simulink model "threelevel_12phase1"  (R2020b)
settings: Solver=FixedStepDiscrete  StartTime=0.0  StopTime=1  FixedStep=Ts_FEA  RelTol=1e-3
model workspace (MAT data in the model file):
  T_10kHz : Simulink.Parameter (value not decoded)
undefined symbols (not defined in the file): Cin, DiscIntNeverNeededParam, ESL, ESR, faif, Jm, kfeed_r, ki_n, kp_n, L, Ld, Line, Lq, ncmd_climb, ncmd_cruise, ncmd_run, ncmd_takeoff, p, Pcmd_climb, Pcmd_cruise, Pcmd_run, Pcmd_takeoff, Rs, Tcmd_run, Tcmd_start, Tcmd_time, time_climb, time_cruise, time_run, time_start, time_takeoff, Ts, Ts_Dead, Ts_FEA, Ts_speedloop, tswitch_climb, tswitch_takeoff, VDC, ws, zero_C1
libraries: powerlib x73, simulink x16, powerlib_meascontrol x16, slpidlib x13
(part 4 of 6)

== matlab function threelevel_12phase1/CurrentLoop/Subsystem/Subsystem/propose method1 ==
  data: PI input; r output; alpha input; beta input; phi input
function r = fcn(PI,alpha,beta,phi)

    M=sqrt(alpha^2+beta^2);
    alp_M  = alpha/M;
    beta_M = beta/M;

    M=1.1547*M;

    if(M<=1/sqrt(3)) 
        M3C= 0.1500*phi*phi*phi+0.0352*phi*phi+0.00783*phi+0.2609;
        M9C=-0.2472*phi*phi*phi-0.0606*phi*phi-0.01287*phi-0.3448;
        M3S= 0.3370*phi*phi+0.6254*phi;
        M9S=-0.0779*phi*phi-0.1659*phi;
    elseif(M<2/3)
        M3C=-3.6560+13.670*M-0.1007*phi-11.930*M*M+0.1374*M*phi+0.1620*phi*phi;
        M9C= 0.4058-3.4580*M+0.1805*phi+3.7340*M*M-0.2433*M*phi-0.2790*phi*phi;
        M3S= 0.7860-2.5180*M-0.6832*phi+2.0240*M*M+2.2250*M*phi+0.3401*phi*phi;
        M9S= 0.0754-0.2625*M+0.4331*phi+0.2243*M*M-1.0250*M*phi-0.0853*phi*phi;
    elseif(M<=0.84)
        M3C= 2.9760-6.4130*M-0.1877*phi+3.2850*M*M+0.2125*M*phi+0.2343*phi*phi;
        M9C=-0.4525-0.6800*M+0.3454*phi+1.4460*M*M-0.3967*M*phi-0.3939*phi*phi;
        M3S= 0.9292-2.4140*M-1.6830*phi+1.5730*M*M+3.5520*M*phi+0.5395*phi*phi;
        M9S=-0.2812+0.7235*M+0.7560*phi-0.4670*M*M-1.4380*M*phi-0.1593*phi*phi; 
    elseif(M<=1.16)
        M3C=-2.1320+5.5280*M-0.3833*phi-3.7000*M*M+0.4197*M*phi+0.2730*phi*phi;
        M9C= 1.0050-3.4350*M+0.5720*phi+2.6570*M*M-0.6220*M*phi-0.4592*phi*phi;
        M3S= 3.3150-7.2060*M-5.4830*phi+3.9060*M*M+8.0500*M*phi+0.4916*phi*phi;
        M9S=-0.9551+2.0770*M+1.5220*phi-1.1270*M*M-2.3370*M*phi-0.1548*phi*phi;
    else
        M3C = 0;
        M9C = 0;
        M3S = 0;
        M9S = 0;
    end

    cos_3 = -3*alp_M + 4*alp_M*alp_M*alp_M;
    cos_9 = -3*cos_3 + 4*cos_3*cos_3*cos_3;
    sin_3 =  3*beta_M - 4*beta_M*beta_M*beta_M;
    sin_9 =  3*sin_3  - 4*sin_3*sin_3*sin_3;
    
    r=M3C*cos_3+ M9C*cos_9+ M3S*sin_3+ M9S*sin_9+PI;
end

== matlab function threelevel_12phase1/CurrentLoop/NTSV_9_nearest ==
  data: Alpha input; Beta input; Ta1 output; Ta2 output; Tb1 output; Tb2 output; Tc1 output; Tc2 output; r input; VecSector1 output
function [Ta1,Ta2,Tb1,Tb2,Tc1,Tc2,VecSector1]  = fcn(Alpha,Beta,r)
temp1=Beta;
temp2=0.8660254*Alpha+Beta*0.5;
temp3=temp2-temp1;%0.8660254*Alpha-0.5beta
%temp1+temp2 0.8660254*Alpha+1.5beta
%temp3+temp2 2*0.8660254*Alpha
%temp1-temp3 -0.8660254*Alpha+1.5beta
VecSector1=3;
VecSector2=1;
VecSector3=0;
if temp2>0
    VecSector1=VecSector1-1;
end
if temp3>0
    VecSector1=VecSector1-1;
end
if temp1<0
    VecSector1=7-VecSector1;
end 
switch VecSector1
    case {1,4}  
       if(abs(temp2)>0.5)
           VecSector2=VecSector2+1;
           if(abs(temp3)<0.5)
               VecSector2=VecSector2+1;
               if(abs(temp1)>0.5)
                   VecSector2=VecSector2+1;
               end
           end
       end
       if(temp1<temp3)
           VecSector3=1;
       else
           VecSector3=2;
       end
    case {2,5}
       if(abs(temp1)>0.5)
           VecSector2=VecSector2+1;
           if(abs(temp2)<0.5)
               VecSector2=VecSector2+1;
               if(abs(temp3)>0.5)
                   VecSector2=VecSector2+1;
               end
           end
       end
       if(temp2+temp3>0)
          VecSector3=1;
       else
           VecSector3=2;
       end 
    case {3,6}
       if(abs(temp3)>0.5)
           VecSector2=VecSector2+1;
           if(abs(temp1)<0.5)
               VecSector2=VecSector2+1;
               if(abs(temp2)>0.5)
                   VecSector2=VecSector2+1;
               end
           end
       end
       if(temp1+temp2>0)
          VecSector3=1;
       else
           VecSector3=2;
       end 
    otherwise
        VecSector1=0;
        VecSector2=0;
end

switch VecSector1
    case 1
        Ta1=temp2;
        Ta2=1;
        Tc1=0;
        Tc2=1-temp2;
        switch VecSector2
            case 1
                Tb1=temp1;
                Tb2=1-temp3;
            case 2
                Tb1=0;
                Tb2=1+temp1-temp3;
            case 3
                Tb1=0.5-temp3;
                Tb2=0.5+temp1;
            case 4
                Tb1=temp1-temp3;
                Tb2=1;
            otherwise
                Tb1=0;
                Tb2=1;
        end
        if(VecSector3==1)
            Ta1=Ta1+Tc2*r;
            Tb2=Tb2+Tc2*r;
            Tc2=Tc2+Tc2*r;
        else
            Ta1=Ta1+Tc2*r;
            Tb1=Tb1+Tc2*r;
            Tc2=Tc2+Tc2*r;
        end
%--------------------------------------------------%
    case 2
        Tb1=temp1;
        Tb2=1;
        Tc1=0;
        Tc2=1-temp1;
        switch VecSector2
            case 1
                Ta1=temp2;
                Ta2=1+temp3;
            case 2
                Ta1=temp2+temp3;
                Ta2=1;
            case 3
                Ta1=0.5+temp3;
                Ta2=0.5+temp2;
            case 4
                Ta1=0;
                Ta2=1+temp2+temp3;
            otherwise
                Ta1=0;
                Ta2=1;
        end
        if(VecSector3==1)
            Ta1=Ta1+Tc2*r;
            Tb1=Tb1+Tc2*r;
            Tc2=Tc2+Tc2*r;
        else
            Ta2=Ta2+Tc2*r;
            Tb1=Tb1+Tc2*r;
            Tc2=Tc2+Tc2*r;
        end
%--------------------------------------------------%
    case 3
        Ta1=0;
        Ta2=1+temp3;
        Tb1=-temp3;
        Tb2=1;
        switch VecSector2
            case 1
                Tc1=-temp2;
                Tc2=1-temp1;
            case 2
                Tc1=0;
                Tc2=1-temp1-temp2;
            case 3
                Tc1=0.5-temp1;
                Tc2=0.5-temp2;
            case 4
                Tc1=-temp1-temp2;
                Tc2=1;
            otherwise
                Tc1=0;
                Tc2=1;
        end
        if(VecSector3==1)
            Tb1=Tb1+Ta2*r;
            Tc2=Tc2+Ta2*r;
            Ta2=Ta2+Ta2*r;
        else
            Tb1=Tb1+Ta2*r;
            Tc1=Tc1+Ta2*r;
            Ta2=Ta2+Ta2*r;
        end
%--------------------------------------------------%
    case 4
        Ta1=0;
        Ta2=1+temp2;
        Tc1=-temp2;
        Tc2=1;
        switch VecSector2
            case 1
                Tb1=-temp3;
                Tb2=1+temp1;
            case 2
                Tb1=temp1-temp3;
                Tb2=1;
            case 3
                Tb1=0.5+temp1;
                Tb2=0.5-temp3;
            case 4
                Tb1=0;
                Tb2=1+temp1-temp3;
            otherwise
                Tb1=0;
                Tb2=1;
        end
        if(VecSector3==1)
            Tb1=Tb1+Ta2*r;
            Tc1=Tc1+Ta2*r;
            Ta2=Ta2+Ta2*r;
        else
            Tb2=Tb2+Ta2*r;
            Tc1=Tc1+Ta2*r;
            Ta2=Ta2+Ta2*r;
        end
%--------------------------------------------------%
    case 5
        Tb1=0;
        Tb2=1+temp1;
        Tc1=-temp1;
        Tc2=1;
        switch VecSector2
            case 1
                Ta1=temp3;
                Ta2=1+temp2;
            case 2
                Ta1=0;
                Ta2=1+temp2+temp3;
            case 3
                Ta1=0.5+temp2;
                Ta2=0.5+temp3;
            case 4
                Ta1=temp2+temp3;
                Ta2=1;
            otherwise
                Ta1=0;
                Ta2=1;
        end
        if(VecSector3==1)
            Ta2=Ta2+Tb2*r;
            Tc1=Tc1+Tb2*r;
            Tb2=Tb2+Tb2*r;
        else
            Ta1=Ta1+Tb2*r;
            Tc1=Tc1+Tb2*r;
            Tb2=Tb2+Tb2*r;
        end
%--------------------------------------------------%
    case 6
        Ta1=temp3;
        Ta2=1;
        Tb1=0;
        Tb2=1-temp3;
        switch VecSector2
            case 1
                Tc1=-temp1;
                Tc2=1-temp2;
            case 2
                Tc1=-temp1-temp2;
                Tc2=1;
            case 3
                Tc1=0.5-temp2;
                Tc2=0.5-temp1;
            case 4
                Tc1=0;
                Tc2=1-temp1-temp2;
            otherwise
                Tc1=0;
                Tc2=1;
        end
        if(VecSector3==1)
            Ta1=Ta1+Tb2*r;
            Tc1=Tc1+Tb2*r;
            Tb2=Tb2+Tb2*r;
        else
            Ta1=Ta1+Tb2*r;
            Tc2=Tc2+Tb2*r;
            Tb2=Tb2+Tb2*r;
        end
%--------------------------------------------------%
    otherwise
        Ta1=0;
        Ta2=1;
        Tb1=0;
        Tb2=1;
        Tc1=0;
        Tc2=1;
end

== matlab function threelevel_12phase1/CurrentLoop/双载波SVPWM2 ==
  data: Alpha input; Beta input; Ta1 output; Ta2 output; Tb1 output; Tb2 output; Tc1 output; Tc2 output; r input; VecSector1 output
function [Ta1,Ta2,Tb1,Tb2,Tc1,Tc2,VecSector1]  = fcn(Alpha,Beta,r)
temp1=Beta;
temp2=0.8660254*Alpha+Beta*0.5;
temp3=temp2-temp1;%0.8660254*Alpha-0.5beta
%temp1+temp2 0.8660254*Alpha+1.5beta
%temp3+temp2 2*0.8660254*Alpha
%temp1-temp3 -0.8660254*Alpha+1.5beta
VecSector1=3;

x=sqrt(3)*Beta;
y=sqrt(3)*(sqrt(3)/2*Alpha+0.5*Beta);
z=sqrt(3)*(-sqrt(3)/2*Alpha+0.5*Beta);

if temp2>0
    VecSector1=VecSector1-1;
end
if temp3>0
    VecSector1=VecSector1-1;
end
if temp1<0
    VecSector1=7-VecSector1;
end 

switch VecSector1
    case 1
        TL=-z;
        TH=x;
        T07=1-TL-TH;
%--------------------------------------------------%
    case 2
        TL=z;
        TH=y;
        T07=1-TL-TH;
%--------------------------------------------------%
    case 3
        TL=x;
        TH=-y;
        T07=1-TL-TH;
%--------------------------------------------------%
    case 4
        TL=-x;
        TH=z;
        T07=1-TL-TH;
%--------------------------------------------------%
    case 5
        TL=-y;
        TH=-z;
        T07=1-TL-TH;
%--------------------------------------------------%
    case 6
        TL=y;
        TH=-x;
        T07=1-TL-TH;
%--------------------------------------------------%
    otherwise
        T07=0;
        TL=0;
        TH=0;
end

T7=T07*(1+r)/2;
Ta=0;
Tb=0;
Tc=0;

switch VecSector1
    case 1
    Ta=TH+TL+T7;
    Tb=TH+T7;
    Tc=T7;
    case  2
    Ta=TH+T7;
    Tb=TH+TL+T7;
    Tc=T7;
    case  3
    Ta=T7;
    Tb=TH+TL+T7;
    Tc=TH+T7;
    case  4
    Ta=T7;
    Tb=TH+T7;
    Tc=TH+TL+T7;
    case  5
    Ta=TH+T7;
    Tb=T7;
    Tc=TH+TL+T7;
    case  6
    Ta=TH+TL+T7;
    Tb=T7;
    Tc=TH+T7;     
end

Ta=Ta*2-1;
Tb=Tb*2-1;
Tc=Tc*2-1;

Ta1=Ta*(Ta>0);
Ta1=1-Ta1;
Ta2=Ta*(Ta<0);
Ta2=Ta2+1;
Ta2=1-Ta2;
Tb1=Tb*(Tb>0);
Tb1=1-Tb1;
Tb2=Tb*(Tb<0);
Tb2=Tb2+1;
Tb2=1-Tb2;
Tc1=Tc*(Tc>0);
Tc1=1-Tc1;
Tc2=Tc*(Tc<0);
Tc2=Tc2+1;
Tc2=1-Tc2;

== matlab function threelevel_12phase1/CurrentLoop/Subsystem2/Subsystem/propose method1 ==
  data: PI input; r output; alpha input; beta input; phi input
function r = fcn(PI,alpha,beta,phi)

    M=sqrt(alpha^2+beta^2);
    alp_M  = alpha/M;
    beta_M = beta/M;

    M=1.1547*M;

    if(M<=1/sqrt(3)) 
        M3C= 0.1500*phi*phi*phi+0.0352*phi*phi+0.00783*phi+0.2609;
        M9C=-0.2472*phi*phi*phi-0.0606*phi*phi-0.01287*phi-0.3448;
        M3S= 0.3370*phi*phi+0.6254*phi;
        M9S=-0.0779*phi*phi-0.1659*phi;
    elseif(M<2/3)
        M3C=-3.6560+13.670*M-0.1007*phi-11.930*M*M+0.1374*M*phi+0.1620*phi*phi;
        M9C= 0.4058-3.4580*M+0.1805*phi+3.7340*M*M-0.2433*M*phi-0.2790*phi*phi;
        M3S= 0.7860-2.5180*M-0.6832*phi+2.0240*M*M+2.2250*M*phi+0.3401*phi*phi;
        M9S= 0.0754-0.2625*M+0.4331*phi+0.2243*M*M-1.0250*M*phi-0.0853*phi*phi;
    elseif(M<=0.84)
        M3C= 2.9760-6.4130*M-0.1877*phi+3.2850*M*M+0.2125*M*phi+0.2343*phi*phi;
        M9C=-0.4525-0.6800*M+0.3454*phi+1.4460*M*M-0.3967*M*phi-0.3939*phi*phi;
        M3S= 0.9292-2.4140*M-1.6830*phi+1.5730*M*M+3.5520*M*phi+0.5395*phi*phi;
        M9S=-0.2812+0.7235*M+0.7560*phi-0.4670*M*M-1.4380*M*phi-0.1593*phi*phi; 
    elseif(M<=1.16)
        M3C=-2.1320+5.5280*M-0.3833*phi-3.7000*M*M+0.4197*M*phi+0.2730*phi*phi;
        M9C= 1.0050-3.4350*M+0.5720*phi+2.6570*M*M-0.6220*M*phi-0.4592*phi*phi;
        M3S= 3.3150-7.2060*M-5.4830*phi+3.9060*M*M+8.0500*M*phi+0.4916*phi*phi;
        M9S=-0.9551+2.0770*M+1.5220*phi-1.1270*M*M-2.3370*M*phi-0.1548*phi*phi;
    else
        M3C = 0;
        M9C = 0;
        M3S = 0;
        M9S = 0;
    end

    cos_3 = -3*alp_M + 4*alp_M*alp_M*alp_M;
    cos_9 = -3*cos_3 + 4*cos_3*cos_3*cos_3;
    sin_3 =  3*beta_M - 4*beta_M*beta_M*beta_M;
    sin_9 =  3*sin_3  - 4*sin_3*sin_3*sin_3;
    
    r=M3C*cos_3+ M9C*cos_9+ M3S*sin_3+ M9S*sin_9+PI;
end

== matlab function threelevel_12phase1/PMSM/MATLAB Function2 ==
  data: I input; Tem output; faif parameter; p parameter; fai_d1 output; fai_d2 output; fai_d3 output; fai_d4 output; fai_q1 output; fai_q2 output; fai_q3 output; fai_q4 output; Temp_L input
function [Tem,fai_d1,fai_d2,fai_d3,fai_d4,fai_q1,fai_q2,fai_q3,fai_q4] = Tem(I,faif,p,Temp_L)

% Temp_fai = Temp_L * I;
Temp_fai=Temp_L;
fai_d1=Temp_fai(1,1)+faif;
fai_d2=Temp_fai(3,1)+faif;
fai_d3=Temp_fai(5,1)+faif;
fai_d4=Temp_fai(7,1)+faif;
fai_q1=Temp_fai(2,1);
fai_q2=Temp_fai(4,1);
fai_q3=Temp_fai(6,1);
fai_q4=Temp_fai(8,1);
Tem1=3/2*p*(fai_d1*I(2,1)-fai_q1*I(1,1));
Tem2=3/2*p*(fai_d2*I(4,1)-fai_q2*I(3,1));
Tem3=3/2*p*(fai_d3*I(6,1)-fai_q3*I(5,1));
Tem4=3/2*p*(fai_d4*I(8,1)-fai_q4*I(7,1));
Tem=Tem1+Tem2+Tem3+Tem4;

== matlab function threelevel_12phase1/CurrentLoop/Subsystem3/NTSV_7_nearest ==
  data: Alpha input; Beta input; Ta1 output; Ta2 output; Tb1 output; Tb2 output; Tc1 output; Tc2 output; r input; r output
function [Ta1,Ta2,Tb1, Tb2,Tc1,Tc2,r]  = fcn(Alpha,Beta,r)
temp1=Beta;
temp2=0.8660254*Alpha+Beta*0.5;
temp3=temp2-temp1;%0.8660254*Alpha-0.5beta
VecSector1=3;
VecSector2=1;
VecSector3=0;
if temp2>0
    VecSector1=VecSector1-1;
end
if temp3>0
    VecSector1=VecSector1-1;
end
if temp1<0
    VecSector1=7-VecSector1;
end 
switch VecSector1
    case {1,4}  
       if(abs(temp2)>0.5)
           VecSector2=VecSector2+1;
           if(abs(temp3)<0.5)
               VecSector2=VecSector2+1;
               if(abs(temp1)>0.5)
                   VecSector2=VecSector2+1;
               end
           end
       end
       if(temp1<temp3)
           VecSector3=1;
       else
           VecSector3=2;
       end
    case {2,5}
       if(abs(temp1)>0.5)
           VecSector2=VecSector2+1;
           if(abs(temp2)<0.5)
               VecSector2=VecSector2+1;
               if(abs(temp3)>0.5)
                   VecSector2=VecSector2+1;
               end
           end
       end
       if(temp2+temp3>0)
          VecSector3=1;
       else
           VecSector3=2;
       end 
    case {3,6}
       if(abs(temp3)>0.5)
           VecSector2=VecSector2+1;
           if(abs(temp1)<0.5)
               VecSector2=VecSector2+1;
               if(abs(temp2)>0.5)
                   VecSector2=VecSector2+1;
               end
           end
       end
       if(temp1+temp2>0)
          VecSector3=1;
       else
           VecSector3=2;
       end 
    otherwise
        VecSector1=0;
        VecSector2=0;
end
switch VecSector1
    case 1
        switch VecSector2
            case 1
                if(VecSector3==1)
                    Ta1=temp3;
                    Ta2=1;
                    Tb1=0;
                    Tb2=1-temp3;
                    Tc1=0;
                    Tc2=1-temp2-temp1;

                    Tb2=Tb2+Ta1*r;
                    Tc2=Tc2+Ta1*r;
                    Ta1=Ta1+Ta1*r;
                elseif(VecSector3==2)
                    Ta1=temp2+temp3;
                    Ta2=1;
                    Tb1=temp1;
                    Tb2=1;
                    Tc1=0;
                    Tc2=1-temp1;

                    Tc2=Tc2+Tb1*r;
                    Ta1=Ta1+Tb1*r;
                    Tb1=Tb1+Tb1*r;
                else
                    Ta1=temp3;
                    Ta2=1;
                    Tb1=0;
                    Tb2=1-temp3;
                    Tc1=0;
                    Tc2=1-temp2-temp1;

                    Tb2=Tb2+Ta1*r;
                    Tc2=Tc2+Ta1*r;
                    Ta1=Ta1+Ta1*r;
                end
            case 2
                Ta1=temp2;
                Ta2=1;
                Tb1=0;
                Tb2=1-temp3+temp1;
                Tc1=0;
                Tc2=1-temp2;
                
                Ta1=Ta1+Tc2*r;
                Tb2=Tb2+Tc2*r;
                Tc2=Tc2+Tc2*r;
            case 3
                if(VecSector3==1)
                    Ta1=temp2+temp3-0.5;
                    Ta2=1;
                    Tb1=0;
                    Tb2=0.5+temp1;
                    Tc1=0;
                    Tc2=0.5-temp1;

                    Ta1=Ta1+Tc2*r;
                    Tb2=Tb2+Tc2*r;
                    Tc2=Tc2+Tc2*r;
                elseif(VecSector3==2)
                    Ta1=0.5+temp3;
                    Ta2=1;
                    Tb1=0.5-temp3;
                    Tb2=1;
                    Tc1=0;
                    Tc2=1.5-temp1-temp2;

                    Ta1=Ta1+Tb1*r;
                    Tc2=Tc2+Tb1*r;
                    Tb1=Tb1+Tb1*r;
                else
                    Ta1=temp2+temp3-0.5;
                    Ta2=1;
                    Tb1=0;
                    Tb2=0.5+temp1;
                    Tc1=0;
                    Tc2=0.5-temp1;

                    Ta1=Ta1+Tc2*r;
                    Tb2=Tb2+Tc2*r;
                    Tc2=Tc2+Tc2*r;
                end
            case 4
                Ta1=temp2;
                Ta2=1;
                Tb1=temp1-temp3;
                Tb2=1;
                Tc1=0;
                Tc2=1-temp2;

                Ta1=Ta1+Tc2*r;
                Tb1=Tb1+Tc2*r;
                Tc2=Tc2+Tc2*r; 
            otherwise
                Ta1=0;
                Ta2=1;
                Tb1=0;
                Tb2=1;
                Tc1=0;
                Tc2=1;
        end
    case 2
        switch VecSector2
            case 1
                if(VecSector3==1)
                    Ta1=temp2;
                    Ta2=1;
                    Tb1=temp1-temp3;
                    Tb2=1;
                    Tc1=0;
                    Tc2=1-temp2;

                    Tb1=Tb1+Ta1*r;
                    Tc2=Tc2+Ta1*r;
                    Ta1=Ta1+Ta1*r;
                elseif(VecSector3==2)
                    Ta1=0;
                    Ta2=1+temp3;
                    Tb1=-temp3;
                    Tb2=1;
                    Tc1=0;
                    Tc2=1-temp2-temp1;
                    
                    Tc2=Tc2+Tb1*r;
                    Ta2=Ta2+Tb1*r;
                    Tb1=Tb1+Tb1*r;
                else
                    Ta1=temp2;
                    Ta2=1;
                    Tb1=temp1-temp3;
                    Tb2=1;
                    Tc1=0;
                    Tc2=1-temp2;

                    Tb1=Tb1+Ta1*r;
                    Tc2=Tc2+Ta1*r;
                    Ta1=Ta1+Ta1*r;
                end
            case 2
                Ta1=temp2+temp3;
                Ta2=1;
                Tb1=temp1;
                Tb2=1;
                Tc1=0;
                Tc2=1-temp1;
                
                Ta1=Ta1+Tc2*r;
                Tb1=Tb1+Tc2*r;
                Tc2=Tc2+Tc2*r;
            case 3
                if(VecSector3==1)
                    Ta1=0.5+temp3;
                    Ta2=1;
                    Tb1=0.5-temp3;
                    Tb2=1;
                    Tc1=0;
                    Tc2=1.5-temp2-temp1;

                    Tb1=Tb1+Ta1*r;
                    Tc2=Tc2+Ta1*r;
                    Ta1=Ta1+Ta1*r;
                elseif(VecSector3==2)
                    Ta1=0;
                    Ta2=0.5+temp2;
                    Tb1=temp1-temp3-0.5;
                    Tb2=1;
                    Tc1=0;
                    Tc2=0.5-temp2;

                    Tb1=Tb1+Tc2*r;
                    Ta2=Ta2+Tc2*r;
                    Tc2=Tc2+Tc2*r;
                else
                    Ta1=0.5+temp3;
                    Ta2=1;
                    Tb1=0.5-temp3;
                    Tb2=1;
                    Tc1=0;
                    Tc2=1.5-temp2-temp1;

                    Tb1=Tb1+Ta1*r;
                    Tc2=Tc2+Ta1*r;
                    Ta1=Ta1+Ta1*r;
                end
            case 4
                Ta1=0;
                Ta2=1+temp2+temp3;
                Tb1=temp1;
                Tb2=1;
                Tc1=0;
                Tc2=1-temp1;
                
                Ta2=Ta2+Tc2*r;
                Tb1=Tb1+Tc2*r;
                Tc2=Tc2+Tc2*r;
            otherwise
                Ta1=0;
                Ta2=1;
                Tb1=0;
                Tb2=1;
                Tc1=0;
                Tc2=1;
        end
    case 3
        switch VecSector2
            case 1
                if(VecSector3==1)
                    Ta1=0;
                    Ta2=1+temp2+temp3;
                    Tb1=temp1;
                    Tb2=1;
                    Tc1=0;
                    Tc2=1-temp1;

                    Ta2=Ta2+Tb1*r;
                    Tc2=Tc2+Tb1*r;
                    Tb1=Tb1+Tb1*r;
                elseif(VecSector3==2)
                    Ta1=0;
                    Ta2=1+temp2;
                    Tb1=temp1-temp3;
                    Tb2=1;
                    Tc1=-temp2;
                    Tc2=1;

                    Ta2=Ta2+Tc1*r;
                    Tb1=Tb1+Tc1*r;
                    Tc1=Tc1+Tc1*r;
                else
                    Ta1=0;
                    Ta2=1+temp2+temp3;
                    Tb1=temp1;
                    Tb2=1;
                    Tc1=0;
                    Tc2=1-temp1;

                    Ta2=Ta2+Tb1*r;
                    Tc2=Tc2+Tb1*r;
                    Tb1=Tb1+Tb1*r;
                end
            case 2
                Ta1=0;
                Ta2=1+temp3;
                Tb1=-temp3;
                Tb2=1;
                Tc1=0;
                Tc2=1-temp2-temp1;

                Tb1=Tb1+Ta2*r;
                Tc2=Tc2+Ta2*r;
                Ta2=Ta2+Ta2*r;
            case 3
                if(VecSector3==1)
                    Ta1=0;
                    Ta2=0.5+temp2;
                    Tb1=-0.5-temp3+temp1;
                    Tb2=1;
                    Tc1=0;
                    Tc2=0.5-temp2;

                    Tb1=Tb1+Ta2*r;
                    Tc2=Tc2+Ta2*r;
                    Ta2=Ta2+Ta2*r;
                elseif(VecSector3==2)
                    Ta1=0;
                    Ta2=1.5+temp2+temp3;
                    Tb1=0.5+temp1;
                    Tb2=1;
                    Tc1=0.5-temp1;
                    Tc2=1;

                    Tb1=Tb1+Tc1*r;
                    Ta2=Ta2+Tc1*r;
                    Tc1=Tc1+Tc1*r;
                else
                    Ta1=0;
                    Ta2=0.5+temp2;
                    Tb1=-0.5-temp3+temp1;
                    Tb2=1;
                    Tc1=0;
                    Tc2=0.5-temp2;

                    Tb1=Tb1+Ta2*r;
                    Tc2=Tc2+Ta2*r;
                    Ta2=Ta2+Ta2*r; 
                end
            case 4
                Ta1=0;
                Ta2=1+temp3;
                Tb1=-temp3;
                Tb2=1;
                Tc1=-temp2-temp1;
                Tc2=1;
                
                Tb1=Tb1+Ta2*r;
                Tc1=Tc1+Ta2*r;
                Ta2=Ta2+Ta2*r;
            otherwise
                Ta1=0;
                Ta2=1;
                Tb1=0;
                Tb2=1;
                Tc1=0;
                Tc2=1;
        end
    case 4
        switch VecSector2
            case 1
                if(VecSector3==2)
                    Ta1=0;
                    Ta2=1+temp3;
                    Tb1=-temp3;
                    Tb2=1;
                    Tc1=-temp2-temp1;
                    Tc2=1;

                    Ta2=Ta2+Tb1*r;
                    Tc1=Tc1+Tb1*r;
                    Tb1=Tb1+Tb1*r;
                elseif(VecSector3==1)
                    Ta1=0;
                    Ta2=1+temp3+temp2;
                    Tb1=0;
                    Tb2=1+temp1;
                    Tc1=-temp1;
                    Tc2=1;

                    Ta2=Ta2+Tc1*r;
                    Tb2=Tb2+Tc1*r;
                    Tc1=Tc1+Tc1*r;
                else
                    Ta1=0;
                    Ta2=1+temp3;
                    Tb1=-temp3;
                    Tb2=1;
                    Tc1=-temp2-temp1;
                    Tc2=1;

                    Ta2=Ta2+Tb1*r;
                    Tc1=Tc1+Tb1*r;
                    Tb1=Tb1+Tb1*r;
                end
            case 2
                Ta1=0;
                Ta2=1+temp2;
                Tb1=temp1-temp3;
                Tb2=1;
                Tc1=-temp2;
                Tc2=1;
                
                Tb1=Tb1+Ta2*r;
                Tc1=Tc1+Ta2*r;
                Ta2=Ta2+Ta2*r;
            case 3
                if(VecSector3==2)
                    Ta1=0;
                    Ta2=1.5+temp2+temp3;
                    Tb1=0.5+temp1;
                    Tb2=1;
                    Tc1=0.5-temp1;
                    Tc2=1;

                    Ta2=Ta2+Tb1*r;
                    Tc1=Tc1+Tb1*r;
                    Tb1=Tb1+Tb1*r;
                elseif(VecSector3==1)
                    Ta1=0;
                    Ta2=0.5+temp3;
                    Tb1=0;
                    Tb2=0.5-temp3;
                    Tc1=-0.5-temp2-temp1;
                    Tc2=1;

                    Tc1=Tc1+Ta2*r;
                    Tb2=Tb2+Ta2*r;
                    Ta2=Ta2+Ta2*r;
                else
                    Ta1=0;
                    Ta2=1.5+temp2+temp3;
                    Tb1=0.5+temp1;
                    Tb2=1;
                    Tc1=0.5-temp1;
                    Tc2=1;

                    Ta2=Ta2+Tb1*r;
                    Tc1=Tc1+Tb1*r;
                    Tb1=Tb1+Tb1*r;
                end
            case 4
                Ta1=0;
                Ta2=1+temp2;
                Tb1=0;
                Tb2=1+temp1-temp3;
                Tc1=-temp2;
                Tc2=1;
                
                Tc1=Tc1+Ta2*r;
                Tb2=Tb2+Ta2*r;
                Ta2=Ta2+Ta2*r;
            otherwise
                Ta1=0;
                Ta2=1;
                Tb1=0;
                Tb2=1;
                Tc1=0;
                Tc2=1;
        end
    case 5
        switch VecSector2
            case 1
                if(VecSector3==2)
                    Ta1=0;
                    Ta2=1+temp2;
                    Tb1=0;
                    Tb2=1-temp3+temp1;
                    Tc1=-temp2;
                    Tc2=1;

                    Ta2=Ta2+Tc1*r;
                    Tb2=Tb2+Tc1*r;
                    Tc1=Tc1+Tc1*r;
                elseif(VecSector3==1)
                    Ta1=temp3;
                    Ta2=1;
                    Tb1=0;
                    Tb2=1-temp3;
                    Tc1=-temp2-temp1;
                    Tc2=1;

                    Tb2=Tb2+Ta1*r;
                    Tc1=Tc1+Ta1*r;
                    Ta1=Ta1+Ta1*r;
                else
                    Ta1=0;
                    Ta2=1+temp2;
                    Tb1=0;
                    Tb2=1-temp3+temp1;
                    Tc1=-temp2;
                    Tc2=1;

                    Ta2=Ta2+Tc1*r;
                    Tb2=Tb2+Tc1*r;
                    Tc1=Tc1+Tc1*r; 
                end
            case 2
                Ta1=0;
                Ta2=1+temp2+temp3;
                Tb1=0;
                Tb2=1+temp1;
                Tc1=-temp1;
                Tc2=1;
                
                Ta2=Ta2+Tb2*r;
                Tc1=Tc1+Tb2*r;
                Tb2=Tb2+Tb2*r;
            case 3
                if(VecSector3==2)
                    Ta1=0;
                    Ta2=0.5+temp3;
                    Tb1=0;
                    Tb2=0.5-temp3;
                    Tc1=-0.5-temp1-temp2;
                    Tc2=1;

                    Ta2=Ta2+Tb2*r;
                    Tc1=Tc1+Tb2*r;
                    Tb2=Tb2+Tb2*r;
                elseif(VecSector3==1)
                    Ta1=0.5+temp2;
                    Ta2=1;
                    Tb1=0;
                    Tb2=1.5-temp3+temp1;
                    Tc1=0.5-temp2;
                    Tc2=1;
 
                    Tc1=Tc1+Ta1*r;
                    Tb2=Tb2+Ta1*r;
                    Ta1=Ta1+Ta1*r;
                else
                    Ta1=0;
                    Ta2=0.5+temp3;
                    Tb1=0;
                    Tb2=0.5-temp3;
                    Tc1=-0.5-temp1-temp2;
                    Tc2=1;

                    Ta2=Ta2+Tb2*r;
                    Tc1=Tc1+Tb2*r;
                    Tb2=Tb2+Tb2*r;
                end
            case 4
                Ta1=temp2+temp3;
                Ta2=1;
                Tb1=0;
                Tb2=1+temp1;
                Tc1=-temp1;
                Tc2=1;
                
                Ta1=Ta1+Tb2*r;
                Tc1=Tc1+Tb2*r;
                Tb2=Tb2+Tb2*r;
            otherwise
                Ta1=0;
                Ta2=1;
                Tb1=0;
                Tb2=1;
                Tc1=0;
                Tc2=1;
        end
    case 6
        switch VecSector2
            case 1
                if(VecSector3==2)
                    Ta1=temp2+temp3;
                    Ta2=1;
                    Tb1=0;
                    Tb2=1+temp1;
                    Tc1=-temp1;
                    Tc2=1;

                    Ta1=Ta1+Tc1*r;
                    Tb2=Tb2+Tc1*r;
                    Tc1=Tc1+Tc1*r;
                elseif(VecSector3==1)
                    Ta1=temp2;
                    Ta2=1;
                    Tb1=0;
                    Tb2=1+temp1-temp3;
                    Tc1=0;
                    Tc2=1-temp2;

                    Tb2=Tb2+Ta1*r;
                    Tc2=Tc2+Ta1*r;
                    Ta1=Ta1+Ta1*r;
                else
                    Ta1=temp2+temp3;
                    Ta2=1;
                    Tb1=0;
                    Tb2=1+temp1;
                    Tc1=-temp1;
                    Tc2=1;

                    Ta1=Ta1+Tc1*r;
                    Tb2=Tb2+Tc1*r;
                    Tc1=Tc1+Tc1*r;
                end
            case 2
                Ta1=temp3;
                Ta2=1;
                Tb1=0;
                Tb2=1-temp3;
                Tc1=-temp2-temp1;
                Tc2=1;
                
                Ta1=Ta1+Tb2*r;
                Tc1=Tc1+Tb2*r;
                Tb2=Tb2+Tb2*r;
            case 3
                if(VecSector3==2)
                    Ta1=0.5+temp2;
                    Ta2=1;
                    Tb1=0;
                    Tb2=1.5+temp1-temp3;
                    Tc1=0.5-temp2;
                    Tc2=1;

                    Ta1=Ta1+Tc1*r;
                    Tb2=Tb2+Tc1*r;
                    Tc1=Tc1+Tc1*r;
                elseif(VecSector3==1)
                    Ta1=-0.5+temp2+temp3;
                    Ta2=1;
                    Tb1=0;
                    Tb2=0.5+temp1;
                    Tc1=0;
                    Tc2=0.5-temp1;

                    Ta1=Ta1+Tb2*r;
                    Tc2=Tc2+Tb2*r;
                    Tb2=Tb2+Tb2*r;
                else
                    Ta1=0.5+temp2;
                    Ta2=1;
                    Tb1=0;
                    Tb2=1.5+temp1-temp3;
                    Tc1=0.5-temp2;
                    Tc2=1;

                    Ta1=Ta1+Tc1*r;
                    Tb2=Tb2+Tc1*r;
                    Tc1=Tc1+Tc1*r;
                end
            case 4
                Ta1=temp3;
                Ta2=1;
                Tb1=0;
                Tb2=1-temp3;
                Tc1=0;
                Tc2=1-temp2-temp1;
                
                Ta1=Ta1+Tb2*r;
                Tc2=Tc2+Tb2*r;
                Tb2=Tb2+Tb2*r;
            otherwise
                Ta1=0;
                Ta2=1;
                Tb1=0;
                Tb2=1;
                Tc1=0;
                Tc2=1;
        end
    otherwise
        Ta1=0;
        Ta2=1;
        Tb1=0;
        Tb2=1;
        Tc1=0;
        Tc2=1;
end

== matlab function threelevel_12phase1/CurrentLoop/Subsystem3/Subsystem/propose method1 ==
  data: PI input; r output; alpha input; beta input; phi input
function r = fcn(PI,alpha,beta,phi)

    M=sqrt(alpha^2+beta^2);
    alp_M  = alpha/M;
    beta_M = beta/M;

    M=1.1547*M;

    if(M<=1/sqrt(3)) 
        M3C= 0.1500*phi*phi*phi+0.0352*phi*phi+0.00783*phi+0.2609;
        M9C=-0.2472*phi*phi*phi-0.0606*phi*phi-0.01287*phi-0.3448;
        M3S= 0.3370*phi*phi+0.6254*phi;
        M9S=-0.0779*phi*phi-0.1659*phi;
    elseif(M<2/3)
        M3C=-3.6560+13.670*M-0.1007*phi-11.930*M*M+0.1374*M*phi+0.1620*phi*phi;
        M9C= 0.4058-3.4580*M+0.1805*phi+3.7340*M*M-0.2433*M*phi-0.2790*phi*phi;
        M3S= 0.7860-2.5180*M-0.6832*phi+2.0240*M*M+2.2250*M*phi+0.3401*phi*phi;
        M9S= 0.0754-0.2625*M+0.4331*phi+0.2243*M*M-1.0250*M*phi-0.0853*phi*phi;
    elseif(M<=0.84)
        M3C= 2.9760-6.4130*M-0.1877*phi+3.2850*M*M+0.2125*M*phi+0.2343*phi*phi;
        M9C=-0.4525-0.6800*M+0.3454*phi+1.4460*M*M-0.3967*M*phi-0.3939*phi*phi;
        M3S= 0.9292-2.4140*M-1.6830*phi+1.5730*M*M+3.5520*M*phi+0.5395*phi*phi;
        M9S=-0.2812+0.7235*M+0.7560*phi-0.4670*M*M-1.4380*M*phi-0.1593*phi*phi; 
    elseif(M<=1.16)
        M3C=-2.1320+5.5280*M-0.3833*phi-3.7000*M*M+0.4197*M*phi+0.2730*phi*phi;
        M9C= 1.0050-3.4350*M+0.5720*phi+2.6570*M*M-0.6220*M*phi-0.4592*phi*phi;
        M3S= 3.3150-7.2060*M-5.4830*phi+3.9060*M*M+8.0500*M*phi+0.4916*phi*phi;
        M9S=-0.9551+2.0770*M+1.5220*phi-1.1270*M*M-2.3370*M*phi-0.1548*phi*phi;
    else
        M3C = 0;
        M9C = 0;
        M3S = 0;
        M9S = 0;
    end

    cos_3 = -3*alp_M + 4*alp_M*alp_M*alp_M;
    cos_9 = -3*cos_3 + 4*cos_3*cos_3*cos_3;
    sin_3 =  3*beta_M - 4*beta_M*beta_M*beta_M;
    sin_9 =  3*sin_3  - 4*sin_3*sin_3*sin_3;
    
    r=M3C*cos_3+ M9C*cos_9+ M3S*sin_3+ M9S*sin_9+PI;
end
